simulink model "lqr_1dof_linear_speed"  (R2017a)
settings: Solver=ode45  StartTime=0.0  StopTime=10  RelTol=1e-3
undefined symbols (not defined in the file): A, B, GoalPos, K, k_p, x0
settings Model: Creator=sansh  LastModifiedBy=rj2318

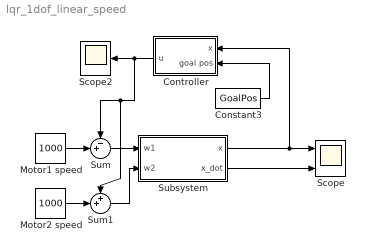
== system lqr_1dof_linear_speed ==
  Constant3 : Constant  Value=GoalPos
  Controller : Subsystem
  Motor1 speed : Constant  Value=1000
  Motor2 speed : Constant  Value=1000
  Scope : Scope  NumInputPorts=2
  Scope2 : Scope
  Subsystem : Subsystem
  Sum : Sum  Inputs=-+|
  Sum1 : Sum  Inputs=++|
  wires:
  Constant3/1 -> Controller/2(goal pos)
  Subsystem/2(x_dot) -> Scope/2
  Subsystem/1(x) -> Controller/1(x), Scope/1
  Sum1/1 -> Subsystem/2(w2)
  Motor2 speed/1 -> Sum1/2
  Controller/1(u) -> Sum1/1, Sum/1, Scope2/1
  Motor1 speed/1 -> Sum/2
  Sum/1 -> Subsystem/1(w1)

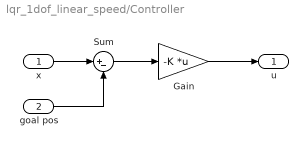
== system lqr_1dof_linear_speed/Controller ==
  x : Inport
  goal pos : Inport  Port=2
  Gain : Gain  Gain=-K  Multiplication=Matrix(K*u)
  Sum : Sum  Inputs=|+-
  u : Outport
  wires:
  x/1 -> Sum/1
  Gain/1 -> u/1
  Sum/1 -> Gain/1
  goal pos/1 -> Sum/2

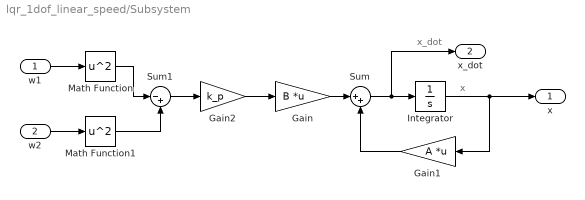
== system lqr_1dof_linear_speed/Subsystem ==
  note: x_dot
  note: x
  w1 : Inport
  w2 : Inport  Port=2
  Gain : Gain  Gain=B  Multiplication=Matrix(K*u)
  Gain1 : Gain  Gain=A  Multiplication=Matrix(K*u)
  Gain2 : Gain  Gain=k_p
  Integrator : Integrator  InitialCondition=x0
  Math Function : Math  Operator=square  SaturateOnIntegerOverflow=on
  Math Function1 : Math  Operator=square  SaturateOnIntegerOverflow=on
  Sum : Sum  Inputs=|++
  Sum1 : Sum  Inputs=|-+
  x : Outport
  x_dot : Outport  Port=2
  wires:
  Gain1/1 -> Sum/2
  Integrator/1 -> Gain1/1, x/1
  Sum/1 -> x_dot/1, Integrator/1
  Gain/1 -> Sum/1
  Math Function/1 -> Sum1/1
  w1/1 -> Math Function/1
  Math Function1/1 -> Sum1/2
  Sum1/1 -> Gain2/1
  w2/1 -> Math Function1/1
  Gain2/1 -> Gain/1
